simulink model "Modelo_GuPu"  (Simulink 10.3)
settings: Solver=ode45  StartTime=0.0  StopTime=1000  MaxStep=0.1  RelTol=1e-6  EnableMultiTasking=on
settings Model: Creator=Marcelo  LastModifiedBy=Fer
settings DataIOCC: SaveOutput=off  SignalLoggingName=sigsOut
settings OptimizationCC: BlockReduction=off  BooleanDataType=off
settings DebuggingCC: SaveWithParameterizedLinksMsg=none  SignalResolutionControl=TryResolveAllWithWarning  MultiTaskDSMMsg=warning  MultiTaskCondExecSysMsg=none
settings HardwareCC: TargetUnknown=on

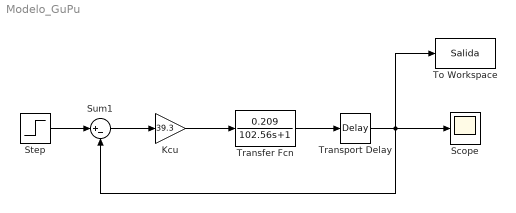
== system Modelo_GuPu ==
  Kcu : Gain  Gain=39.3
  Scope : Scope
  Step : Step  Time=50  Before=1  SampleTime=0
  Sum1 : Sum  Inputs=|+-  InputSameDT=on  SaturateOnIntegerOverflow=on  OutDataTypeStr=Inherit: Same as first input
  To Workspace : ToWorkspace  VariableName=Salida
  Transfer Fcn : TransferFcn  Numerator=[0.209]  Denominator=[102.56 1]
  Transport Delay : TransportDelay  DelayTime=21.3
  wires:
  Transfer Fcn/1 -> Transport Delay/1
  Transport Delay/1 -> To Workspace/1, Scope/1, Sum1/2
  Kcu/1 -> Transfer Fcn/1
  Sum1/1 -> Kcu/1
  Step/1 -> Sum1/1
